simulink model "model_qube_test"  (R2025a)
settings: Solver=FixedStepDiscrete  StartTime=0.0  StopTime=inf  FixedStep=0.02  RelTol=1e-3  EnableMultiTasking=on
values from neighbouring files (symbols this model uses):
  Npred = 5    [my_mpc_codegen.m]
  Ts = 0.02    [my_mpc_codegen.m]
undefined symbols (not defined in the file or in its folder): HIL
libraries: quarc_library x6, dspbuff3 x2
settings Model: ExtModeTrigDuration=10000  Creator=khanh  LastModifiedBy=khanh
settings SolverCC: AlgebraicLoopSolver=TrustRegion  PositivePriorityOrder=on
settings DataIOCC: ReturnWorkspaceOutputs=off
settings DebuggingCC: UnconnectedInputMsg=warning  UnconnectedOutputMsg=warning  UnconnectedLineMsg=warning  ArithmeticOperatorsInVariantConditions=warning
settings ModelReferenceCC: EnableRefExpFcnMdlSchedulingChecks=on
settings SFSimCC: SimUseLocalCustomCode=off  CustomCodeUndefinedFunction=UseInterfaceOnly
settings RTWCC: SystemTargetFile=quarc_win64.tlc  TemplateMakefile=quarc_default_tmf  RTWUseLocalCustomCode=off  CustomSource=C:\Users\khanh\dev\python\projects\casadi_codegen\basics\sfunction_builder\my_solver.c  Toolchain=QUARC win64 | nmake (64-bit Windows)  BuildConfiguration=Faster Runs  GPUComputeCapability=3.5  Description=QUARC Win64 Target Using Toolchain
settings RTWCC: CustomInclude=|
  | C:\Users\khanh\dev\python\projects\casadi_codegen\basics\sfunction_builder
  | C:\Users\khanh\dev\matlab\casadi-3.7.1-windows64-matlab2018b\include
  | C:\Users\khanh\dev\matlab\casadi-3.7.1-windows64-matlab2018b
settings RTWCC: CustomLibrary=|
  | C:\Users\khanh\dev\matlab\casadi-3.7.1-windows64-matlab2018b\ipopt.lib
  | C:\Users\khanh\dev\matlab\casadi-3.7.1-windows64-matlab2018b\lapack.lib
settings CodeAppCC: StateflowObjectComments=on
settings STFCustomTargetCC: SystemTargetFile=quarc_win64.tlc  TargetLangStandard=C99 (ISO)  MultiwordLength=2048.0  DynamicStringBufferSize=256.0  ConcurrentExecutionCompliant=on  UseToolchainInfoCompliant=on
settings GRTTargetCC: ExtMode=on  ExtModeMexFile=quarc_comm  ParMdlRefBuildCompliant=off  CompOptLevelCompliant=off  CombineOutputUpdateFcns=off  MatFileLogging=off  CPPClassGenCompliant=off  GRTInterface=on
settings ConfigComp: CovMetricSettings=dswe

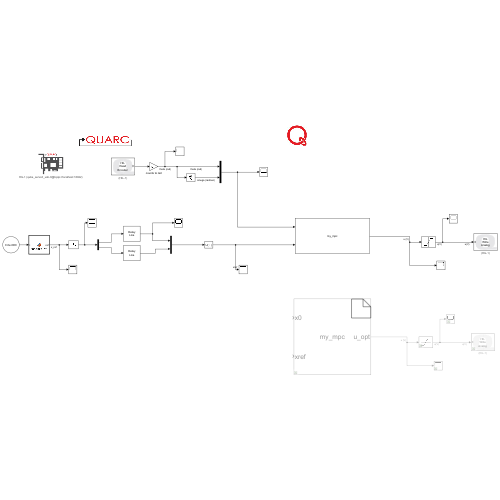
[thumbnail: Simulink's stored preview of the top-level diagram]
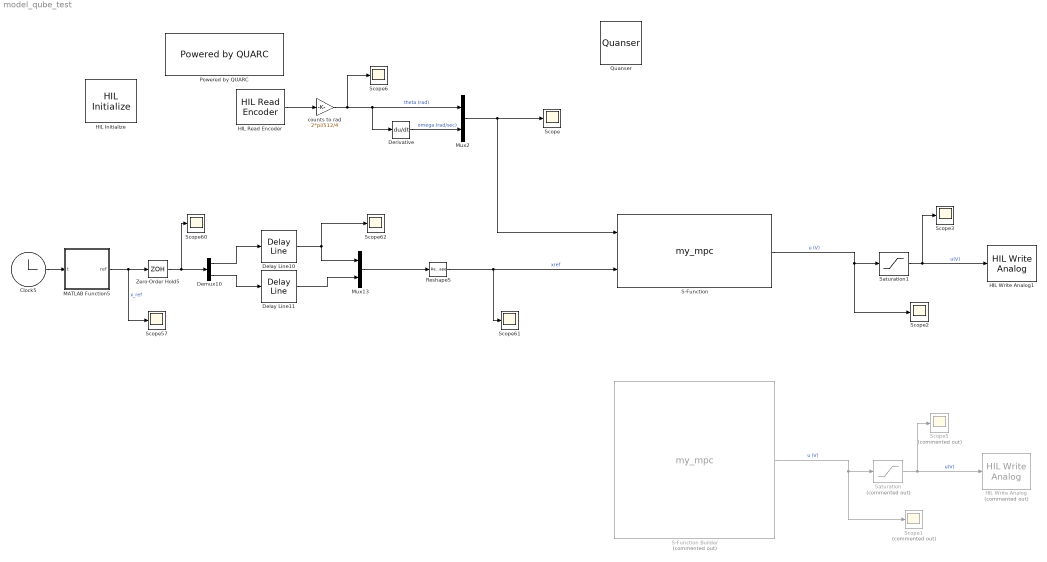
== system model_qube_test ==
  Clock5 : Clock
  Delay Line10 : dspbuff3/Delay Line  siz=Npred+1  ic=0  directfeed=off  enable_output=off  hold_output=off  OutputFrames=off
  Delay Line11 : dspbuff3/Delay Line  siz=Npred+1  ic=0  directfeed=off  enable_output=off  hold_output=off  OutputFrames=off
  Demux10 : Demux  Outputs=2
  Derivative : Derivative
  HIL Initialize : quarc_library/Data Acquisition/Generic/Configuration/HIL Initialize  object_name=HIL-1  board_type=qube_servo3_usb  board_number=0@tcpip://localhost:18922  board_options=deadband_compensation=0.3;pwm_en=0;enc0_velocity=3.0;enc1_velocity=3.0;min_diode_compensation=0.3;max_diode_compensation=1.5  exclusive=off  active=on  hardware_clocks=[0]  clock_modes=[]  initial_clock_frequencies=[]  set_clock_params_at_start=off  set_clock_params_at_switch_in=off  set_clock_frequencies_at_start=off  set_clock_frequencies_at_switch_in=off  analog_input_channels=[0]  analog_input_configurations=[]  analog_input_maximums=3  analog_input_minimums=-3  set_analog_input_params_at_start=off  set_analog_input_params_at_switch_in=off  analog_output_channels=[0]  analog_output_maximums=15  analog_output_minimums=-15  initial_analog_outputs=[0]  final_analog_outputs=[0]  watchdog_analog_outputs=0  set_analog_output_params_at_start=off  set_analog_output_params_at_switch_in=off  set_analog_outputs_at_start=on  set_analog_outputs_at_switch_in=off  set_analog_outputs_at_terminate=on  set_analog_outputs_at_switch_out=off  set_analog_outputs_on_watchdog=on  digital_input_channels=[]  digital_output_channels=[0]  digital_output_configuration=[]  initial_digital_outputs=[1]  final_digital_outputs=[0]  watchdog_digital_outputs=[0]  set_digital_output_params_at_start=off  set_digital_output_params_at_switch_in=off  set_digital_outputs_at_start=on  set_digital_outputs_at_switch_in=off  set_digital_outputs_at_terminate=on  set_digital_outputs_at_switch_out=off  set_digital_outputs_on_watchdog=on  encoder_channels=[0:1]  quadrature=[4]  encoder_filter_frequency=[]  initial_encoder_counts=[0]  set_encoder_params_at_start=off  set_encoder_params_at_switch_in=off  set_encoder_counts_at_start=on  set_encoder_counts_at_switch_in=off  pwm_channels=[]  pwm_modes=[0]  pwm_frequency=23195  pwm_configuration=[1]  pwm_alignment=[0]  pwm_polarity=[1]  pwm_leading_deadband=[0]  pwm_trailing_deadband=[0]  initial_pwm_outputs=[0]  final_pwm_outputs=[0]  watchdog_pwm_outputs=[]  set_pwm_params_at_start=off  set_pwm_params_at_switch_in=off  set_pwm_outputs_at_start=off  set_pwm_outputs_at_switch_in=off  set_pwm_outputs_at_terminate=off  set_pwm_outputs_at_switch_out=off  set_pwm_outputs_on_watchdog=off  other_output_channels=[11000:11002]  initial_other_outputs=[0 1 0]  final_other_outputs=[1 0 0]  watchdog_other_outputs=[0 0 1]  set_other_outputs_at_start=on  set_other_outputs_at_switch_in=off  set_other_outputs_at_terminate=on  set_other_outputs_at_switch_out=off  set_other_outputs_on_watchdog=on
  HIL Read Encoder : quarc_library/Data Acquisition/Generic/Immediate I//O/HIL Read Encoder  object_name=HIL-1  channels=0  sample_time=qc_get_step_size  active=on  vector_output=off  data_type_mode=Inherit via back propagation  data_type=double
  HIL Write Analog : quarc_library/Data Acquisition/Generic/Immediate I//O/HIL Write Analog  Commented=on  object_name=HIL-1  channels=0  sample_time=-1  active=off  vector_input=off
  HIL Write Analog1 : quarc_library/Data Acquisition/Generic/Immediate I//O/HIL Write Analog  object_name=HIL-1  channels=0  sample_time=-1  active=off  vector_input=off
  MATLAB Function5 : MATLAB Function  TreatAsAtomicUnit=on
  Mux13 : Mux  Inputs=2
  Mux2 : Mux  Inputs=2
  Powered by QUARC : quarc_library/Logos/Powered by QUARC
  Quanser : quarc_library/Logos/Quanser
  Reshape5 : Reshape
  S-Function : S-Function  FunctionName=my_mpc  SFunctionModules=my_mpc_wrapper.cpp my_solver  SFunctionDeploymentMode=off  EnableBusSupport=off
  S-Function Builder : S-Function  Commented=on  FunctionName=my_mpc  SFunctionModules=my_mpc_wrapper.cpp my_solver  SFunctionDeploymentMode=off  EnableBusSupport=off  mask(S-Function Builder){}
      mask help: Simulink:masks:SFunctionBuilder_MD
      mask init:
      | val = [[.9  0.75 0.75 1 1 .9 .9 1]',[1 1 0.75 0.75 .9 .9 1 .9]'];try , sys = get_param(gcb,'SfunBuilderFcnName');if isempty(sys), sys = get_param(gcb,'FunctionName'); end,catch, sys = get_param(gcb,'FunctionName'); end
      settings: CopyFcn=set_param(gcbh,'LinkStatus','none')  OpenFcn=sfunctionwizard(gcbh)
      mask Display:
      | plot(val(:,1),val(:,2))
      | disp(sys)
      | port_label('input',1,sprintf('%s', 'x0'),'interpreter','tex')
      | port_label('input',2,sprintf('%s', 'xref'),'interpreter','tex')
      | port_label('output',1,sprintf('%s', 'u\_opt'),'interpreter','tex')
  Saturation : Saturate  Commented=on  UpperLimit=10  LowerLimit=-10
  Saturation1 : Saturate  UpperLimit=10  LowerLimit=-10
  Scope{,2..3,6,57,60..62} (8 alike) : Scope
      Scope settings: ActiveDisplayYMinimum=-1  ActiveDisplayYMaximum=1
      Scope2 settings: ActiveDisplayYMinimum=-12.5  ActiveDisplayYMaximum=12.5  DataLoggingVariableName=ScopeData4
      Scope3 settings: ActiveDisplayYMinimum=-5.44917  ActiveDisplayYMaximum=5.44917  DataLoggingVariableName=ScopeData6
      Scope57 settings: ActiveDisplayYMinimum=-0.98175  ActiveDisplayYMaximum=0.98175  DataLoggingVariableName=ScopeData5
      Scope6 settings: ActiveDisplayYMinimum=-1  ActiveDisplayYMaximum=1  DataLoggingVariableName=ScopeData2
      Scope60 settings: ActiveDisplayYMinimum=-0.98175  ActiveDisplayYMaximum=0.98175  DataLoggingVariableName=ScopeData8
      Scope61 settings: ActiveDisplayYMinimum=-0.98174770424681035  ActiveDisplayYMaximum=0.98174770424681035  DataLoggingVariableName=ScopeData9
      Scope62 settings: ActiveDisplayYMinimum=-0.98175  ActiveDisplayYMaximum=0.98175  DataLoggingVariableName=ScopeData10
  Scope1 : Scope  Commented=on
      settings: ActiveDisplayYMinimum=-12.5  ActiveDisplayYMaximum=12.5
  Scope5 : Scope  Commented=on
      settings: ActiveDisplayYMinimum=-5.44917  ActiveDisplayYMaximum=5.44917  DataLoggingVariableName=ScopeData3
  Zero-Order Hold5 : ZeroOrderHold  SampleTime=Ts
  counts to rad : Gain  Gain=2*pi/512/4
  wires:
  HIL Read Encoder/1 -> counts to rad/1
  counts to rad/1 -> Scope6/1, Mux2/1, Derivative/1  "theta (rad)"
  Mux2/1 -> S-Function/1, Scope/1
  Derivative/1 -> Mux2/2  "omega (rad/sec)"
  Demux10/2 -> Delay Line11/1
  Reshape5/1 -> S-Function/2, Scope61/1  "xref"
  Clock5/1 -> MATLAB Function5/1(t)
  Delay Line11/1 -> Mux13/2
  Zero-Order Hold5/1 -> Demux10/1, Scope60/1
  Mux13/1 -> Reshape5/1
  Delay Line10/1 -> Mux13/1, Scope62/1
  Demux10/1 -> Delay Line10/1
  MATLAB Function5/1(ref) -> Scope57/1, Zero-Order Hold5/1  "x_ref"
  S-Function Builder/1 -> Scope1/1, Saturation/1  "u (V)"
  Saturation/1 -> HIL Write Analog/1, Scope5/1  "u(V)"
  Saturation1/1 -> HIL Write Analog1/1, Scope3/1  "u(V)"
  S-Function/1 -> Scope2/1, Saturation1/1  "u (V)"

== matlab function model_qube_test/MATLAB Function5 ==
  data: t input; ref output
function ref = generate_ref(t)
    amp = pi/4;
    freq = 0.5;
    ref1 = -amp * square(2*pi*freq*t);
    ref2 = 0;
    ref = [ref1; ref2];
end
